simulink model "testHomingGenerator"  (R2016b)
settings: Solver=FixedStepAuto  StartTime=0.0  StopTime=10.0  FixedStep=0.02  RelTol=1e-3
libraries: VariousLibrary x3, PositionSmoothener x1
settings Model: DataDictionary=ModelDictionary.sldd  Creator=march  LastModifiedBy=march

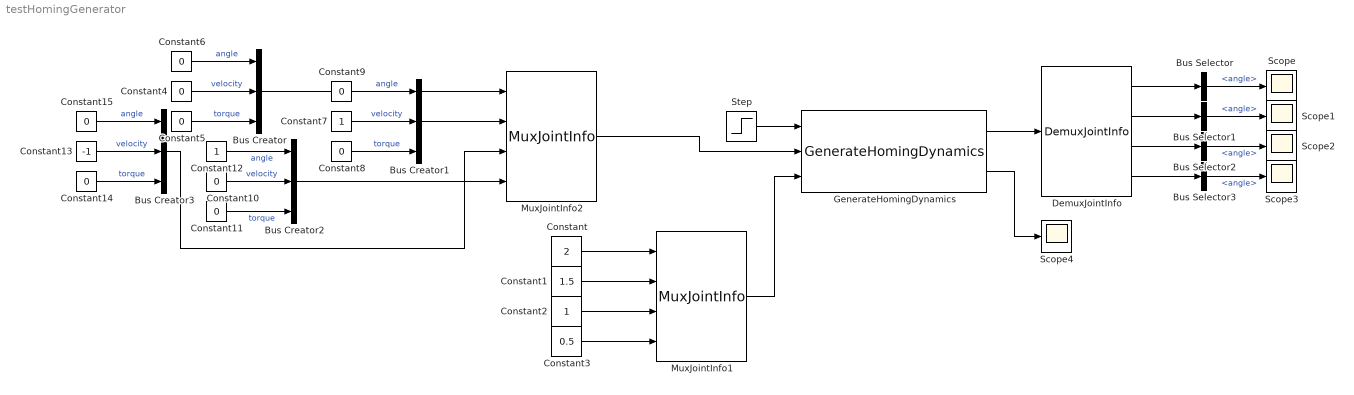
== system testHomingGenerator ==
  Bus Creator{,1..3} (4 alike) : BusCreator  Inputs=3  OutDataTypeStr=Bus: JointDynamics  NonVirtualBus=on
  Bus Selector{,1..3} (4 alike) : BusSelector  OutputSignals=angle
  Constant : Constant  Value=2
  Constant1 : Constant  Value=1.5
  Constant{4..6,8..11,14..15} (9 alike) : Constant  Value=0
  Constant12 : Constant
  Constant13 : Constant  Value=-1
  Constant2 : Constant
  Constant3 : Constant  Value=0.5
  Constant7 : Constant
  DemuxJointInfo : VariousLibrary/DemuxJointInfo
  GenerateHomingDynamics : PositionSmoothener/GenerateHomingDynamics
  MuxJointInfo1 : VariousLibrary/MuxJointInfo
  MuxJointInfo2 : VariousLibrary/MuxJointInfo
  Scope{,1..4} (5 alike) : Scope
  Step : Step  SampleTime=0
  wires:
  Constant/1 -> MuxJointInfo1/1
  Constant3/1 -> MuxJointInfo1/4
  Constant2/1 -> MuxJointInfo1/3
  Constant1/1 -> MuxJointInfo1/2
  Constant6/1 -> Bus Creator/1  "angle"
  Constant5/1 -> Bus Creator/3  "torque"
  Constant4/1 -> Bus Creator/2  "velocity"
  Bus Creator/1 -> MuxJointInfo2/1
  Constant9/1 -> Bus Creator1/1  "angle"
  Constant8/1 -> Bus Creator1/3  "torque"
  Constant7/1 -> Bus Creator1/2  "velocity"
  Bus Creator1/1 -> MuxJointInfo2/2
  Constant12/1 -> Bus Creator2/1  "angle"
  Constant11/1 -> Bus Creator2/3  "torque"
  Constant10/1 -> Bus Creator2/2  "velocity"
  Bus Creator2/1 -> MuxJointInfo2/4
  Constant15/1 -> Bus Creator3/1  "angle"
  Constant14/1 -> Bus Creator3/3  "torque"
  Constant13/1 -> Bus Creator3/2  "velocity"
  Bus Creator3/1 -> MuxJointInfo2/3
  MuxJointInfo2/1 -> GenerateHomingDynamics/2
  MuxJointInfo1/1 -> GenerateHomingDynamics/3
  Step/1 -> GenerateHomingDynamics/1
  GenerateHomingDynamics/1 -> DemuxJointInfo/1
  DemuxJointInfo/1 -> Bus Selector/1
  Bus Selector/1 -> Scope/1  "<angle>"
  DemuxJointInfo/2 -> Bus Selector1/1
  Bus Selector1/1 -> Scope1/1  "<angle>"
  Bus Selector2/1 -> Scope2/1  "<angle>"
  Bus Selector3/1 -> Scope3/1  "<angle>"
  DemuxJointInfo/3 -> Bus Selector2/1
  DemuxJointInfo/4 -> Bus Selector3/1
  GenerateHomingDynamics/2 -> Scope4/1
